simulink model "PI_vectorial_ideal"  (R2021b)
settings: Solver=VariableStepAuto  StartTime=0.0  StopTime=30  RelTol=1e-3
undefined symbols (not defined in the file): K, ki
settings Model: Creator=parra  LastModifiedBy=parra

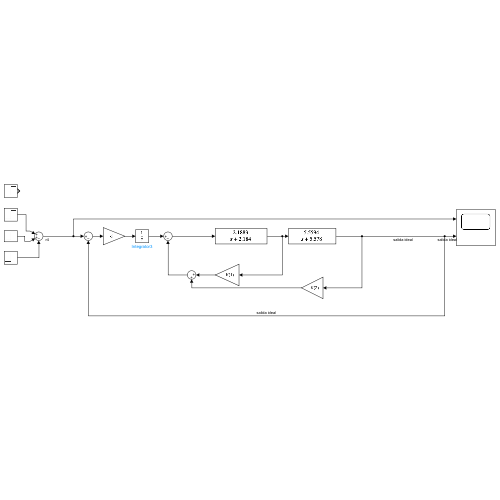
[thumbnail: Simulink's stored preview of the top-level diagram]
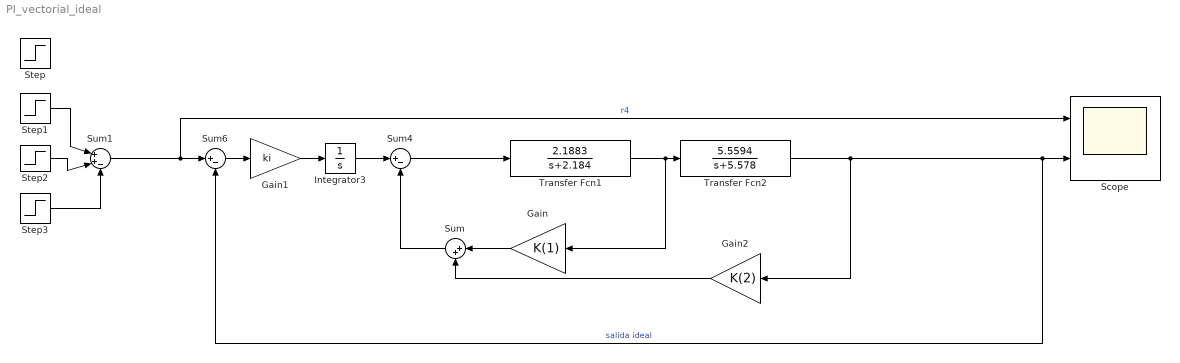
== system PI_vectorial_ideal ==
  Gain : Gain  Gain=K(1)
  Gain1 : Gain  Gain=ki
  Gain2 : Gain  Gain=K(2)
  Integrator3 : Integrator
  Scope : Scope  NumInputPorts=2
  Step : Step  Time=10  Before=0.5  SampleTime=0.01
  Step1 : Step  Time=10  SampleTime=0.01
  Step2 : Step  Time=20  SampleTime=0.01
  Step3 : Step  Time=30  After=2  SampleTime=0.01
  Sum : Sum  Inputs=|++
  Sum1 : Sum  Inputs=|++-
  Sum4 : Sum  Inputs=|+-
  Sum6 : Sum  Inputs=|+-
  Transfer Fcn1 : TransferFcn  Numerator=[2.1883]  Denominator=[1 2.184]
  Transfer Fcn2 : TransferFcn  Numerator=[5.5594]  Denominator=[1 5.578]
  wires:
  Transfer Fcn2/1 -> Scope/2, Sum6/2, Gain2/1  "salida ideal"
  Sum4/1 -> Transfer Fcn1/1
  Integrator3/1 -> Sum4/1
  Gain1/1 -> Integrator3/1
  Sum6/1 -> Gain1/1
  Transfer Fcn1/1 -> Gain/1, Transfer Fcn2/1
  Gain2/1 -> Sum/2
  Gain/1 -> Sum/1
  Sum/1 -> Sum4/2
  Sum1/1 -> Scope/1, Sum6/1  "r4"
  Step1/1 -> Sum1/1
  Step3/1 -> Sum1/3
  Step2/1 -> Sum1/2
